simulink model "psbhvdc"  (Simulink 6.0)
settings: Solver=FixedStepDiscrete  SolverMode=SingleTasking  StartTime=0.0  StopTime=0.8  RelTol=1e-4
InitFcn:
  | powericon('psbinitsys',bdroot);
undefined symbols (not defined in the file or in its folder): D1, Delta
libraries: powerlib2 x36, powerlib_extras x7
settings Model: Creator=patrice  LastModifiedBy=batserve  ExtModeTrigMode=oneshot  ExtModeArmWhenConnect=off  ExtModeAutoUpdateStatusClock=off
settings DataIOCC: LimitDataPoints=off  SaveOutput=off  TimeSaveName=t  SignalLoggingName=sigsOut
settings OptimizationCC: BlockReduction=off  BooleanDataType=off
settings DebuggingCC: CheckExecutionContextPreStartOutputMsg=on  CheckExecutionContextRuntimeOutputMsg=on  SolverPrmCheckMsg=none
settings HardwareCC: TargetUnknown=on
settings RTWCC: TemplateMakefile=grt_unix.tmf

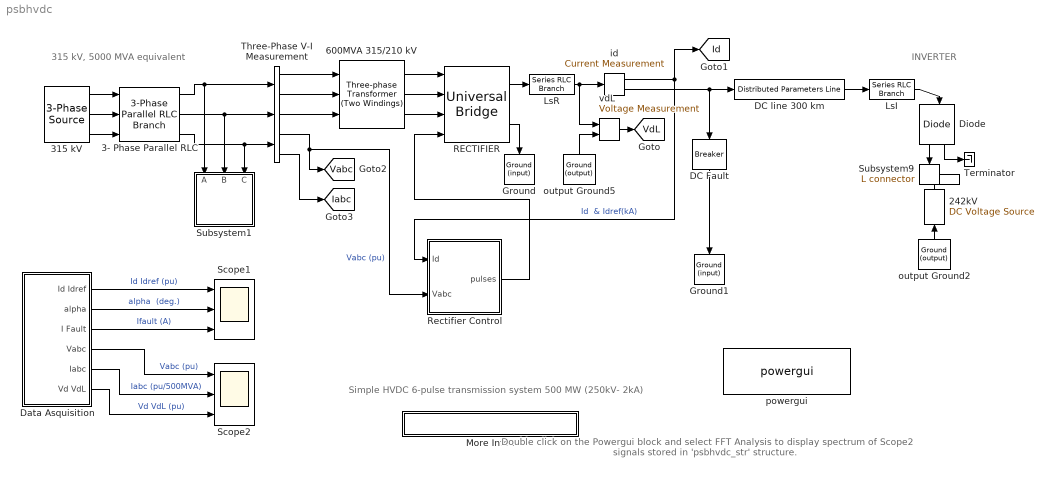
== system psbhvdc ==
  note: INVERTER
  note: Simple HVDC 6-pulse transmission system
      | 500 MW (250kV- 2kA)
  note: 315 kV, 5000 MVA equivalent
  note: Double click on the Powergui block
      | and select  FFT Analysis to display
      |  spectrum of Scope2  signals stored
      | in 'psbhvdc_str' structure.
  242kV : powerlib2/Electrical Sources/DC Voltage Source  Tag=PoWeRsYsTeMbLoCk  Description=source block  Orientation=up  V=242000  mesure=None  PSBOutputType=1
  3- Phase Parallel RLC : powerlib2/Elements/3-Phase Parallel RLC Branch  R=12.41  L=23.264e-3  C=0
  315 kV : powerlib2/Electrical Sources/3-Phase Source  Tag=PoWeRsYsTeMbLoCk  V=315e3  Phi=0  F=60  InternalConnection=Yg  RLoff=off  R=0  L=46.671e-3  Psc=0  Vbase=0  XRratio=0  PSBOutputType=111
  600MVA 315/210 kV : powerlib2/Elements/Three-phase Transformer (Two Windings)  Tag=PoWeRsYsTeMbLoCk  nominal=[ 600e6 60 ]  type1=Yg  params1="[ 315e3*0.97 0.0015  0.0 ]"  type2=Delta (D1)  params2=[ 210e3 0.0015 0.12]  ynsat=off  rmag=500  lm=500  sat="[ 0,0  ;  0.005,1.2  ;  1.0,1.4 ]"  hyst=off  matfile='hysteresis'  sif=off  phi0=[ 0.8 , -0.8 , 0.7 ]  initialslopes=[+1 +1 +1]  mesure=None  PSBOutputType=1111
  DC Fault : powerlib2/Elements/Breaker  Tag=PoWeRsYsTeMbLoCk  Orientation=down  a=0.1  c=0  rs=inf  cs=0  times=[ 0.5 0.51 ]  Ts=0  comext=off  mesure=Branch current  PSBOutputType=1
  DC line 300 km : powerlib2/Elements/Distributed Parameters Line  Tag=PoWeRsYsTeMbLoCk  n=1  f=60  r=0.015  l=0.792e-3  c=14.4e-9  lgt=300  x1=[0 0 0 0; 0.0001244 0 0 0; 0.0002488 0 0 0; 0.0003733 0 0 0; 0.0004977 0 0 0; 0.0006221 0 0 0]  x2=[0 0 0 0; 0.0001244 0 0 0; 0.0002488 0 0 0; 0.0003733 0 0 0; 0.0004977 0 0 0; 0.0006221 0 0 0]  x3=[0 0 0 0; 0.0001244 0 0 0; 0.0002488 0 0 0; 0.0003733 0 0 0; 0.0004977 0 0 0; 0.0006221 0 0 0]  x4=[0 0 0 0; 0.0001244 0 0 0; 0.0002488 0 0 0; 0.0003733 0 0 0; 0.0004977 0 0 0; 0.0006221 0 0 0]  x5=0  mesure=None  PSBOutputType=111111111111111111111111111111
  Data Asquisition : Subsystem
  Diode : powerlib2/Power Electronics/Diode  Tag=PoWeRsYsTeMbLoCk  Orientation=down  Ron=0.01  Lon=0  Vf=0.8  IC=0  Rs=1000  Cs=0.05e-6  PSBOutputType=10
  Ground : powerlib2/Connectors/Ground (input)  Tag=PoWeRsYsTeMbLoCk  Orientation=down
  Ground1 : powerlib2/Connectors/Ground (input)  Tag=PoWeRsYsTeMbLoCk  Orientation=down
  LsI : powerlib2/Elements/Series RLC Branch  Tag=PoWeRsYsTeMbLoCk  a=.5  b=.5  c=inf  mesure=None  PSBOutputType=1
  "LsR " : powerlib2/Elements/Series RLC Branch  Tag=PoWeRsYsTeMbLoCk  a=.5  b=.5  c=inf  mesure=None  PSBOutputType=1
  More Info1 : Subsystem
      mask Display: disp('? : Double click here for more info')
  RECTIFIER : powerlib2/Power Electronics/Universal Bridge  Tag=PoWeRsYsTeMbLoCk  arms=3  confi=ABC as input terminals  injcc=2000  cf=50e-9  device=Thyristors  Ron=1e-3  Lon=0  VFs="[  0.8  0.8  ]"  Vf=0  gtoparameters=[ 10e-6 , 20e-6 ]  igbtparameters=[ 1e-6 , 2e-6 ]  mesure=UAB UBC UCA UDC voltages  PSBOutputType=111
  Rectifier Control : Subsystem
  Scope1 : Scope  NumInputPorts=3
      settings: TimeRange=0.8  YMin=-0.25~0~-500  YMax=2~170~6000  DataFormat=Array
  Scope2 : Scope  NumInputPorts=3
      settings: TimeRange=0.8  YMin=-1.5~-3~-1.5  YMax=1.5~3~2  SaveName=psbhvdc_str
  Subsystem1 : Subsystem  Orientation=down
      mask Display: disp('AC filters \n(320 Mvar)')
  Subsystem9 : powerlib2/Connectors/L connector  Tag=PoWeRsYsTeMbLoCk  Orientation=down
  Terminator : Terminator
  Three-Phase V-I Measurement : powerlib2/Measurements/Three-Phase V-I Measurement  Tag=PoWeRsYsTeMmEaSuReMeNt  VChoice=phase-to-ground  ualv=off  labelV=V1  Vpu=on  Vbase=315e3  IChoice=yes  ualc=off  labelC=I1  Ppu=on  Pbase=500e6  OutputType=Magnitude  PhasorSimulation=off  PSBequivalent=0  PSBOutputType=11100
  id : powerlib2/Measurements/Current Measurement  Tag=PoWeRsYsTeMmEaSuReMeNt  PhasorSimulation=off  OutputType=Complex  PSBOutputType=01  PSBequivalent=0
  output Ground2 : powerlib2/Connectors/Ground (output)  Tag=PoWeRsYsTeMbLoCk  Orientation=up  PSBOutputType=1
  output Ground5 : powerlib2/Connectors/Ground (output)  Tag=PoWeRsYsTeMbLoCk  Orientation=up  PSBOutputType=1
  powergui : powerlib2/powergui  Frange=[0:2:500]  Ylog=off  Xlog=off  save=off  variable=ZData  structure=psbhvdc_str  ZoomFFT=on  StartTime=0.8-2/60  cycles=2  DisplayStyle=off  fundamental=60  FreqAxis=on  MaxFrequency=2000  frequencyindice=1  frequencyindicesteady=1  RmsSteady=1  display=off  Ts=1/360/64  methode=off  frequency=60  echomessages=off
  vdL : powerlib2/Measurements/Voltage Measurement  Tag=PoWeRsYsTeMmEaSuReMeNt  PhasorSimulation=off  OutputType=Complex  PSBOutputType=0  PSBequivalent=0
  tag scope: Iabc=global, Id=global, Vabc=global, VdL=global
  wires:
  RECTIFIER/1 -> "LsR "/1
  RECTIFIER/2 -> Ground/1
  600MVA 315/210 kV/1 -> RECTIFIER/1
  600MVA 315/210 kV/2 -> RECTIFIER/2
  600MVA 315/210 kV/3 -> RECTIFIER/3
  Rectifier Control/1(pulses) -> RECTIFIER/4
  Three-Phase V-I Measurement/1 -> 600MVA 315/210 kV/1
  Three-Phase V-I Measurement/2 -> 600MVA 315/210 kV/2
  Three-Phase V-I Measurement/3 -> 600MVA 315/210 kV/3
  DC line 300 km/1 -> LsI/1
  id/2 -> DC line 300 km/1, DC Fault/1
  "LsR "/1 -> id/1, vdL/1
  output Ground5/1 -> vdL/2
  Data Asquisition/6(Vd VdL) -> Scope2/3  "Vd VdL (pu)"
  id/1 -> Rectifier Control/1(Id), [Id]  "Id  & Idref(kA)"
  Data Asquisition/1("Id Idref ") -> Scope1/1  "Id Idref (pu)"
  DC Fault/1 -> Ground1/1
  Data Asquisition/3(I Fault) -> Scope1/3  "Ifault (A)"
  output Ground2/1 -> 242kV/1
  LsI/1 -> Diode/1
  Diode/1 -> Subsystem9/1
  242kV/1 -> Subsystem9/Enable
  Three-Phase V-I Measurement/4 -> Rectifier Control/2(Vabc), [Vabc]  "Vabc (pu)"
  Diode/2 -> Terminator/1
  3- Phase Parallel RLC/2 -> Subsystem1/2(B), Three-Phase V-I Measurement/2
  vdL/1 -> [VdL]
  Data Asquisition/2(alpha) -> Scope1/2  "alpha  (deg.)"
  3- Phase Parallel RLC/1 -> Three-Phase V-I Measurement/1, Subsystem1/1(A)
  3- Phase Parallel RLC/3 -> Three-Phase V-I Measurement/3, Subsystem1/3(C)
  Data Asquisition/4(Vabc) -> Scope2/1  "Vabc (pu)"
  Data Asquisition/5(Iabc) -> Scope2/2  "Iabc (pu/500MVA)"
  Three-Phase V-I Measurement/5 -> [Iabc]
  315 kV/1 -> 3- Phase Parallel RLC/1
  315 kV/2 -> 3- Phase Parallel RLC/2
  315 kV/3 -> 3- Phase Parallel RLC/3

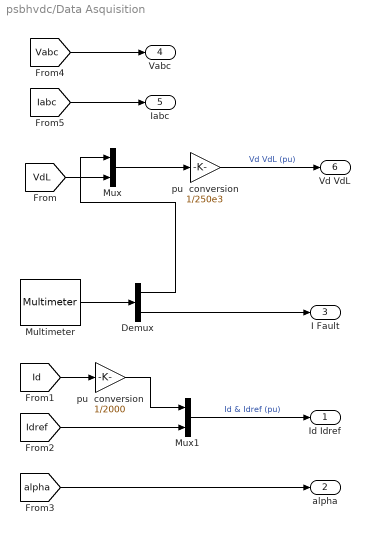
== system psbhvdc/Data Asquisition ==
  Demux : Demux  Outputs=2
  Multimeter : powerlib2/Measurements/Multimeter  Tag=PoWeRsYsTeMmEaSuReMeNt  PhasorSimulation=off  OutputType=Magnitude  sel=[4 5]  L=5  Gain=[1 1]  yselected={'Udc: RECTIFIER','Ib: DC Fault'};  PSBOutputType=1  PSBequivalent=0  AxesSetting=[0,0.1,-100,100]  Display=0  SavedBlockNames={}
  Mux : Mux  Inputs=2
  Mux1 : Mux  Inputs=2
  pu  conversion : Gain  Gain=1/2000  SaturateOnIntegerOverflow=on
  "pu  conversion " : Gain  Gain=1/250e3  SaturateOnIntegerOverflow=on
  "Id Idref " : Outport
  alpha : Outport  Port=2
  I Fault : Outport  Port=3
  Vabc : Outport  Port=4
  Iabc : Outport  Port=5
  Vd VdL : Outport  Port=6
  wires:
  Mux/1 -> "pu  conversion "/1
  [VdL] -> Mux/2
  [Id] -> pu  conversion/1
  Mux1/1 -> "Id Idref "/1  "Id & Idref (pu)"
  [Idref] -> Mux1/2
  Multimeter/1 -> Demux/1
  Demux/2 -> I Fault/1
  Demux/1 -> Mux/1
  [alpha] -> alpha/1
  [Vabc] -> Vabc/1
  [Iabc] -> Iabc/1
  "pu  conversion "/1 -> Vd VdL/1  "Vd VdL (pu)"
  pu  conversion/1 -> Mux1/1

== system psbhvdc/More Info1 ==
  note: Note: In oder to appreciate the speed improvemnt obtained with discretisation, you may try continuous simulation mode after completing this demo.
      |          The discrete system is approximately 6 times faster.
  note: Notice that the system is discretized (sample time 1/360/64 = 43.4 us). Setting, the sample time in to zero, will change to continuous integration for the power system .
  note: Frequency analysis of AC and DC voltages and currents
  note: In order to alllow further signal processing, signals displayed on Scope2 have been saved in a variable named 'psbvdc_str' ( structure with time').
      | These signals are : AC voltages (input 1) , AC currents (input 2) and DC voltages on rectifier and line side of the smoothing reactor (input 3).
      |
      | Open the Powergui and select  'FFT Analysis'. In the FFT window select structure 'psbhvdc_str'. The 0 - 2000 Hz FFT will be performed on  a 2-cycle window starting
      | at t = 0.8 - 2/60 (last 2 cycles of recording). Select input  labeled 'Iabc' . By default Phase a current (signal number 1) is selected. Press on 'Display' and observe
      |  the frequency spectrum of AC current. Harmonic currents (order 6n+/-1 , n = 1,2,3, ...for a 6-pulse converter) are displayed in % of the fundamental component .
      | If you analyze AC voltage (input Vabc) you shoud notice that the highest harmonics generated by the converter (5th and 7th) are filtered out by the two filters tuned at
      | the 5th and 7th harmonics.  Finally, select input labeled 'Vd VdL (pu)' and then input 1 or input 2.  You will obtain harmonic content (order 6n) of  the DC voltage Vd
      | (rectifier side) or VdL (line side) expressed in % of the DC component.
  note: G. Sybille (Hydro-Quebec)
  note: At t = 0.57 s, the regulator is released and it starts to regulate the DC current again. The steady-state 1 pu current is reached at t = 0.75 s.
  note: 0.57 < t < 0.8 s
  note: At t = 0.55 s, the alpha angle is forced by the protection system (not simulated) to reach 165 degrees when the Forced_alpha input of the current regulator goes high (1).
      | The rectifier thus passes in inverter mode and sends the energy stored in the line back to the 345 kV network.
      | As a result, the arc current producing the fault rapidly decreases . The fault is cleared at t = 0.555 s when the fault current zero crossing is reached.
  note: 0.55 < t <0.57 s
  note: At t = 0.5 s, a DC fault is applied on the line. The fault current ( trace 3) increases to 5 kA and the Id current increases to to 2 pu (4 kA) in 10 ms.
      | Then,  the fast regulator action lowers the current back to its reference value of 1 pu..
  note: 0.5 < t < 0.55 s
  note: 0.3 < t < 0.5 s
  note: At t = 0.3 s, the reference current is increased from  0.5 pu (1 kA) to the nominal current  1pu (2 kA). The current regulator  responds in approximately 0.1 s (6 cycles).
      | The alpha angle decreases from 30 degrees to 15 degrees.
  note: Trace 1 shows the the reference current (magenta) and the measured Id current (yellow). The reference current is set to 0.5 pu (1 kA). The DC current starts from zero
      | and reaches a steady-state in 0.1 s. Trace 2 shows the alpha firing angle required to obtain 0.5 pu of current (30 degrees).
  note: 0 < t < 0.3 s
  note: The system is programmed to start and  reach a steady state.  Then, a step is applied on the reference current to observe the dynamic response of the regulator.
      | Finally a DC fault is applied on the line.
      |
      | Start the simulation and observe the following events on  Scope1 :
  note: CIRCUIT DESCRIPTION
  note: This demonstration  illustrates steady-state and transient performance
      | of a simple 500 MW (250 kV-2kA) HVDC transmission system
  note: A 500 MW (250 kV, 2 kA) DC linterconnexion is used to transmit power from a 315 kV, 5000 MVA AC network. The network is simulated by a LLR damped equivalent
      | (impedance angle of 80 degrees at 60 Hz and 3rd harmonic). The converter transformer  and the rectifier are modelled respectively with the Universal Transformer
      | and Universal Bridge blocks The converter is a 6-pulse rectifier. It is connected to a 300 km distributed parameter line through a 0.5 H smoothing reactor LsR.
      | The inverter is simulated by a simple DC voltage source in series with a diode (to force unidirectional conduction) and smoothing reactor LsI.
      | The reactive power required by the converter is provided by a set of filters (C bank plus 5th, 7th and high pass filters; total 320 Mvar).
      | Open the AC filter subsystem to see the filter toplogy.  A circuit breaker allows to apply a DC line fault on the rectifier side.
      |
      | The control system uses two main blocks: the Synchronized 6-pulse generator of the Extras/Control library and a PI Curent Regulator.
      | Voltages sent to the synchronization system are filtered by 2nd order band pass filters. The whole control system is discretized (Sample time = 1/360/64 = 43.4 us).
      |
      | THe DC line current at the output of the rectifier is compared with a reference. The PI regulator tries to keep the error at zero and outputs the alpha firing angle required
      | by the synchronizing unit. Inputs 3 and 4 of the current regulator allow to bypass the regulator action and to impose the alpha firing angle
  note: DEMONSTRATION

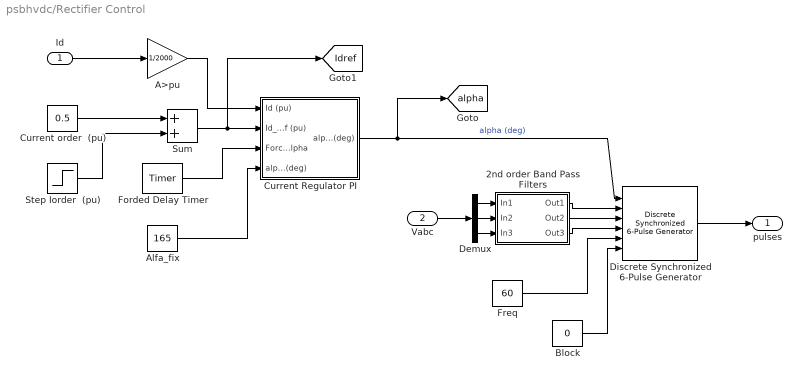
== system psbhvdc/Rectifier Control ==
  Id : Inport  Port=1  LatchInput=off
  Vabc : Inport  Port=2  LatchInput=off
  2nd order Band Pass Filters : Subsystem
      mask Display:
      | disp(' Fo=60 Hz\n\n
      | BW=30 Hz')
  A>pu : Gain  Gain=1/2000  SaturateOnIntegerOverflow=on
  Alfa_fix : Constant  Value=165
  Block : Constant  Value=0
  Current Regulator PI : Subsystem
  Current order  (pu) : Constant  Value=0.5
  Demux : Demux  Outputs=3
  Discrete Synchronized 6-Pulse Generator : powerlib_extras/Discrete  Control Blocks/Discrete Synchronized 6-Pulse Generator  pwidth=70  Double_Pulse=off  Ts=1/360/64
  Forded Delay Timer : powerlib_extras/Control  Blocks/Timer  t=[ 0.55 0.57]  e="[1 0  ]"
  Freq : Constant  Value=60
  "Step Iorder  (pu)  " : Step  Time=0.3  After=0.6  SampleTime=0  ZeroCross=off
  Sum : Sum  SaturateOnIntegerOverflow=on  InputSameDT=on
  pulses : Outport
  tag scope: Idref=global, alpha=global
  wires:
  Demux/1 -> 2nd order Band Pass Filters/1(In1)
  Demux/3 -> 2nd order Band Pass Filters/3(In3)
  Demux/2 -> 2nd order Band Pass Filters/2(In2)
  2nd order Band Pass Filters/2(Out2) -> Discrete Synchronized 6-Pulse Generator/3
  2nd order Band Pass Filters/1(Out1) -> Discrete Synchronized 6-Pulse Generator/2
  2nd order Band Pass Filters/3(Out3) -> Discrete Synchronized 6-Pulse Generator/4
  Block/1 -> Discrete Synchronized 6-Pulse Generator/6
  Freq/1 -> Discrete Synchronized 6-Pulse Generator/5
  Vabc/1 -> Demux/1
  Discrete Synchronized 6-Pulse Generator/1 -> pulses/1
  Current order  (pu)/1 -> Sum/1
  "Step Iorder  (pu)  "/1 -> Sum/2
  Sum/1 -> Current Regulator PI/2(Id_ref (pu)), [Idref]
  A>pu/1 -> Current Regulator PI/1(Id (pu))
  Current Regulator PI/1(alpha (deg)) -> Discrete Synchronized 6-Pulse Generator/1, [alpha]  "alpha (deg)"
  Alfa_fix/1 -> Current Regulator PI/4(alpha_fix(deg))
  Forded Delay Timer/1 -> Current Regulator PI/3(Forced_alpha)
  Id/1 -> A>pu/1

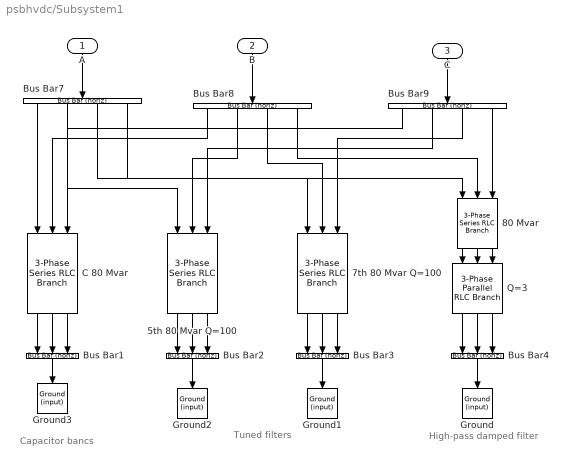
== system psbhvdc/Subsystem1 ==
  note: High-pass
      | damped filter
  note: Tuned filters
  note: Capacitor bancs
  A : Inport  Orientation=down  Port=1  LatchInput=off
  B : Inport  Orientation=down  Port=2  LatchInput=off
  C : Inport  Orientation=down  Port=3  LatchInput=off
  "5th 80 Mvar Q=100 " : powerlib2/Elements/3-Phase Series RLC Branch   Orientation=down  R=2.48  L=131.5e-3  C=2.14e-6
  7th 80 Mvar Q=100 : powerlib2/Elements/3-Phase Series RLC Branch   Orientation=down  R=1.77  L=67.1e-3  C=2.14e-6
  80 Mvar : powerlib2/Elements/3-Phase Series RLC Branch   Orientation=down  R=0  L=0  C=2.14e-6
  Bus Bar{1..4} (4 alike) : powerlib2/Connectors/Bus Bar (horiz)  Tag=PoWeRsYsTeMbLoCk  Orientation=down  entrees=3  sorties=1  PSBOutputType=1111111111111111111111111111111111111111111111111111111111111111111111111
  Bus Bar7 : powerlib2/Connectors/Bus Bar (horiz)  Tag=PoWeRsYsTeMbLoCk  Orientation=down  entrees=1  sorties=4  PSBOutputType=1111111111111111111111111111111111111111111111111111111111111111111111111
  Bus Bar8 : powerlib2/Connectors/Bus Bar (horiz)  Tag=PoWeRsYsTeMbLoCk  Orientation=down  entrees=1  sorties=4  PSBOutputType=1111111111111111111111111111111111111111111111111111111111111111111111111
  Bus Bar9 : powerlib2/Connectors/Bus Bar (horiz)  Tag=PoWeRsYsTeMbLoCk  Orientation=down  entrees=1  sorties=4  PSBOutputType=1111111111111111111111111111111111111111111111111111111111111111111111111
  C 80 Mvar : powerlib2/Elements/3-Phase Series RLC Branch   Orientation=down  R=0  L=0  C=2.14e-6
  Ground{,1..3} (4 alike) : powerlib2/Connectors/Ground (input)  Tag=PoWeRsYsTeMbLoCk  Orientation=down
  Q=3 : powerlib2/Elements/3-Phase Parallel RLC Branch  Orientation=down  R=225.6  L=27.2e-3  C=0
  wires:
  80 Mvar/3 -> Q=3/3
  80 Mvar/2 -> Q=3/2
  80 Mvar/1 -> Q=3/1
  Bus Bar4/1 -> Ground/1
  Bus Bar3/1 -> Ground1/1
  Bus Bar2/1 -> Ground2/1
  Bus Bar9/2 -> "5th 80 Mvar Q=100 "/3
  Bus Bar7/2 -> "5th 80 Mvar Q=100 "/1
  Bus Bar8/2 -> "5th 80 Mvar Q=100 "/2
  "5th 80 Mvar Q=100 "/3 -> Bus Bar2/3
  "5th 80 Mvar Q=100 "/2 -> Bus Bar2/2
  "5th 80 Mvar Q=100 "/1 -> Bus Bar2/1
  Bus Bar1/1 -> Ground3/1
  C 80 Mvar/3 -> Bus Bar1/3
  C 80 Mvar/2 -> Bus Bar1/2
  C 80 Mvar/1 -> Bus Bar1/1
  Bus Bar9/4 -> 80 Mvar/3
  Bus Bar9/3 -> 7th 80 Mvar Q=100/3
  Bus Bar9/1 -> C 80 Mvar/3
  Bus Bar7/4 -> 80 Mvar/1
  Bus Bar7/3 -> 7th 80 Mvar Q=100/1
  Bus Bar8/4 -> 80 Mvar/2
  Bus Bar8/3 -> 7th 80 Mvar Q=100/2
  Bus Bar8/1 -> C 80 Mvar/2
  Bus Bar7/1 -> C 80 Mvar/1
  Q=3/3 -> Bus Bar4/3
  Q=3/2 -> Bus Bar4/2
  Q=3/1 -> Bus Bar4/1
  7th 80 Mvar Q=100/3 -> Bus Bar3/3
  7th 80 Mvar Q=100/2 -> Bus Bar3/2
  7th 80 Mvar Q=100/1 -> Bus Bar3/1
  C/1 -> Bus Bar9/1
  B/1 -> Bus Bar8/1
  A/1 -> Bus Bar7/1

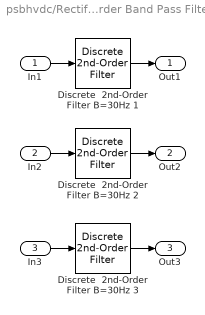
== system psbhvdc/Rectifier Control/2nd order Band Pass Filters ==
  In1 : Inport  Port=1  LatchInput=off
  In2 : Inport  Port=2  LatchInput=off
  In3 : Inport  Port=3  LatchInput=off
  Discrete  2nd-Order Filter B=30Hz 1 : powerlib_extras/Discrete  Control Blocks/Discrete  2nd-Order Filter  FilterType=Bandpass  Fo=60  Zeta=0.25  Ts=1/360/64  Initialize=on  Vac_Init=[0.8 -25 60]  Vdc_Init=-0.4  PlotResponse=off  param1=[1 500 0.1]
  Discrete  2nd-Order Filter B=30Hz 2 : powerlib_extras/Discrete  Control Blocks/Discrete  2nd-Order Filter  FilterType=Bandpass  Fo=60  Zeta=0.25  Ts=1/360/64  Initialize=on  Vac_Init=[0.8 -25 60]  Vdc_Init=-0.4  PlotResponse=off  param1=[1 500 0.1]
  Discrete  2nd-Order Filter B=30Hz 3 : powerlib_extras/Discrete  Control Blocks/Discrete  2nd-Order Filter  FilterType=Bandpass  Fo=60  Zeta=0.25  Ts=1/360/64  Initialize=on  Vac_Init=[0.8 -25 60]  Vdc_Init=-0.4  PlotResponse=off  param1=[1 500 0.1]
  Out1 : Outport
  Out2 : Outport  Port=2
  Out3 : Outport  Port=3
  wires:
  Discrete  2nd-Order Filter B=30Hz 1/1 -> Out1/1
  In1/1 -> Discrete  2nd-Order Filter B=30Hz 1/1
  In2/1 -> Discrete  2nd-Order Filter B=30Hz 2/1
  In3/1 -> Discrete  2nd-Order Filter B=30Hz 3/1
  Discrete  2nd-Order Filter B=30Hz 2/1 -> Out2/1
  Discrete  2nd-Order Filter B=30Hz 3/1 -> Out3/1

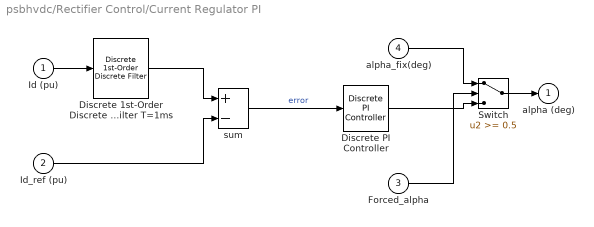
== system psbhvdc/Rectifier Control/Current Regulator PI ==
  Id (pu) : Inport  Port=1  LatchInput=off
  Id_ref (pu) : Inport  Port=2  LatchInput=off
  Forced_alpha : Inport  Port=3  LatchInput=off
  alpha_fix(deg) : Inport  Port=4  LatchInput=off
  Discrete 1st-Order Discrete Filter T=1ms : powerlib_extras/Discrete  Control Blocks/Discrete 1st-Order Discrete Filter  FilterType=Lowpass  Tc=1e-3  Ts=1/360/64  Initialize=off  Vac_Init=[0.8 -25 60]  Vdc_Init=-0.4  PlotResponse=off  param1=[1 500 0.1]
  Discrete PI Controller : powerlib_extras/Discrete  Control Blocks/Discrete PI Controller  Kp=65  Ki=5000  Par_Limits=[165 5]  Init=90  Ts=1/360/64
  Switch : Switch  Threshold=0.5  ZeroCross=off  InputSameDT=on
  sum : Sum  Inputs=+-  SaturateOnIntegerOverflow=on  InputSameDT=on
  alpha (deg) : Outport  InitialOutput=0
  wires:
  Id_ref (pu)/1 -> sum/2
  Discrete 1st-Order Discrete Filter T=1ms/1 -> sum/1
  Id (pu)/1 -> Discrete 1st-Order Discrete Filter T=1ms/1
  sum/1 -> Discrete PI Controller/1  "error"
  Forced_alpha/1 -> Switch/2
  Switch/1 -> alpha (deg)/1
  alpha_fix(deg)/1 -> Switch/1
  Discrete PI Controller/1 -> Switch/3
